simulink model "ex4_2"  (R2018b)
settings: Solver=VariableStepAuto  StartTime=0.0  StopTime=200.0  RelTol=1e-3
settings Model: Creator=HYJ  LastModifiedBy=HYJ
settings SFSimCC: SimUseLocalCustomCode=off
settings RTWCC: RTWUseLocalCustomCode=off

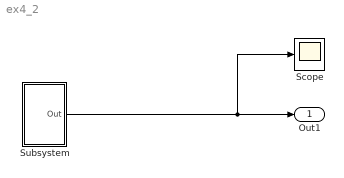
== system ex4_2 ==
  Scope : Scope
  Subsystem : Subsystem  mask{k=5, a1=1, a2=1, m=70, g=10}
  Out1 : Outport
  wires:
  Subsystem/1(Out) -> Scope/1, Out1/1

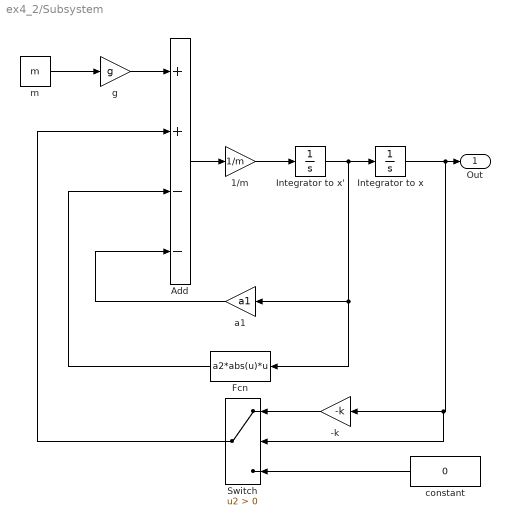
== system ex4_2/Subsystem ==
  " Integrator to x" : Integrator
  -k : Gain  Gain=-k
  1/m : Gain  Gain=1/m
  Add : Sum  Inputs=++--
  Fcn : Fcn  Expr=a2*abs(u)*u
  Integrator to x' : Integrator
  Switch : Switch  Criteria=u2 > Threshold
  a1 : Gain  Gain=a1
  constant : Constant  Value=0
  g : Gain  Gain=g
  m : Constant  Value=m
  Out : Outport
  wires:
  a1/1 -> Add/4
  m/1 -> g/1
  Fcn/1 -> Add/3
  Switch/1 -> Add/2
  Add/1 -> 1/m/1
  1/m/1 -> Integrator to x'/1
  " Integrator to x"/1 -> Switch/2, -k/1, Out/1
  constant/1 -> Switch/3
  g/1 -> Add/1
  -k/1 -> Switch/1
  Integrator to x'/1 -> Fcn/1, a1/1, " Integrator to x"/1
